simulink model "Simulation"  (R2025b)
settings: Solver=VariableStepAuto  StartTime=0.0  StopTime=10.0  RelTol=1e-3
values from neighbouring files (symbols this model uses):
  x0 = [1 1 1 1]'    [main.m]
settings Model: Creator=flof  LastModifiedBy=2712f

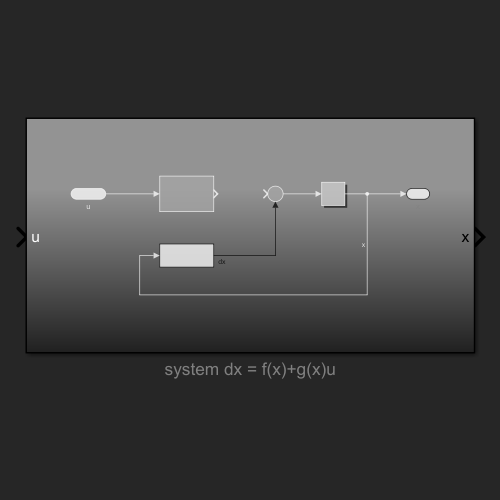
[thumbnail: Simulink's stored preview of the top-level diagram]
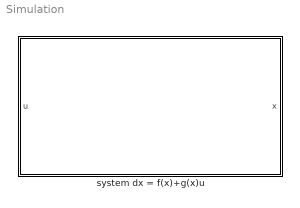
== system Simulation ==
  system dx = f(x)+g(x)u : Subsystem

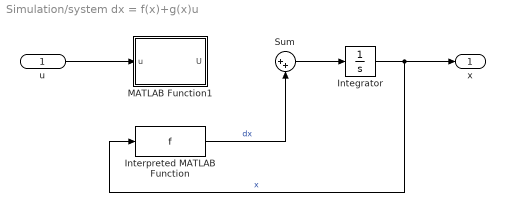
== system Simulation/system dx = f(x)+g(x)u ==
  u : Inport
  Integrator : Integrator  InitialCondition=x0
  Interpreted MATLAB Function : MATLABFcn  MATLABFcn=f
  MATLAB Function1 : MATLAB Function  TreatAsAtomicUnit=on
  Sum : Sum  Inputs=|++
  x : Outport
  wires:
  Integrator/1 -> Interpreted MATLAB Function/1, x/1  "x"
  u/1 -> MATLAB Function1/1(u)
  Sum/1 -> Integrator/1
  Interpreted MATLAB Function/1 -> Sum/2  "dx"

== matlab function Simulation/system dx = f(x)+g(x)u/MATLAB Function1 ==
  data: u input; U output
function U = fcn(u)

    %U = M(x((n+1):(end)))\u;
    U = u;
end
